simulink model "simulatneously"  (R2015b)
settings: Solver=VariableStepAuto  StartTime=0.0  StopTime=5  RelTol=1e-3
libraries: powerlib x36, powerlib_meascontrol x7, powerlib_extras x7
settings Model: Creator=fujitsu  LastModifiedBy=fujitsu

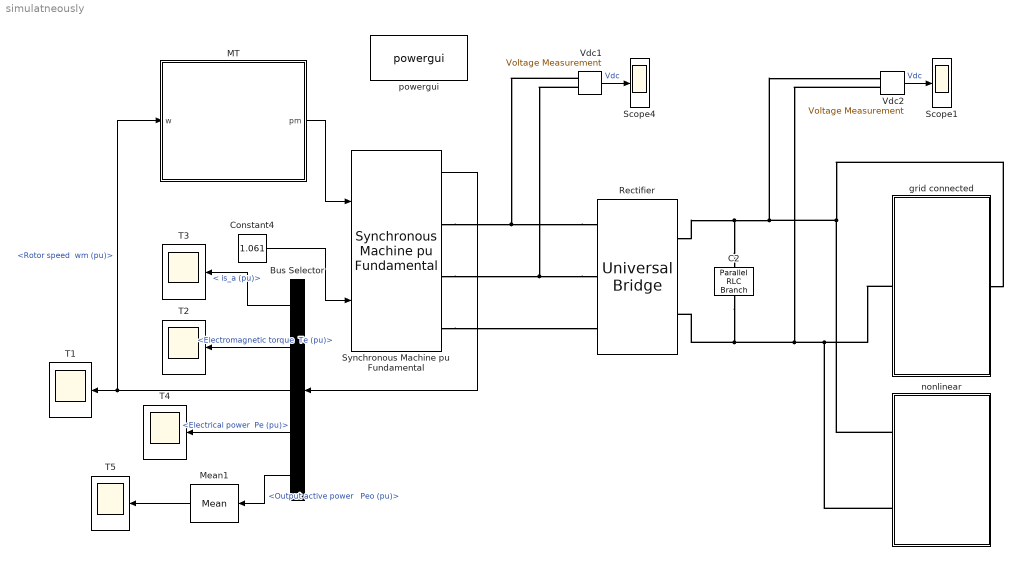
== system simulatneously ==
  Bus Selector : BusSelector  OutputSignals="Stator current. is_a (pu),Mechanical.Electromagnetic torque  Te (pu),Mechanical.Rotor speed  wm (pu),Mechanical.Electrical power  Pe (pu),Output active power   Peo (pu)"
  C2 : powerlib/Elements/Parallel RLC Branch  LConnTagsString=a  RConnTagsString=__new0  BranchType=C  Resistance=inf  Inductance=inf  SetiL0=off  InitialCurrent=0  Capacitance=5000e-05  Setx0=off  InitialVoltage=0  Measurements=None
  Constant4 : Constant  Value=1.061
  MT : Subsystem
  Mean1 : powerlib_meascontrol/Measurements/Mean  Freq=50  Vinit=0  Ts=50e-6
  Rectifier : powerlib/Power Electronics/Universal Bridge  Arms=3  SnubberResistance=50  SnubberCapacitance=0.1e-6  Device=Diodes  Ron=1e-3  Lon=0  ForwardVoltages="[  0.8  0.8  ]"  ForwardVoltage=.7  GTOparameters=[ 10e-6 , 20e-6 ]  IGBTparameters=[ 1e-6 , 2e-6 ]  Measurements=Device currents  Measurements_2=None  converterType=Rectifier
  Scope1 : Scope
  Scope4 : Scope
  Synchronous Machine pu Fundamental : powerlib/Machines/Synchronous Machine pu Fundamental  PresetModel=No  MechanicalLoad=Mechanical power Pm  ShowDetailedParameters=on  RotorType=Salient-pole  Units=per unit fundamental parameters  MeasurementBus=off  NominalParameters="[ 65e3  500 1600]"  Stator="[ 0.2503  0.114  0.6875  0.6875 ]"  Field="[ 1  10e15/(100*pi)]"  Dampers2=[0.0652, 0.5134, 0.0287, 0.2553, 7.765e-3, 0.9167 ]  Dampers1="[ 1.17E-02  0.182  1.97E-02  0.384 ]"  Mechanical=[ 6 0 2]  PolePairs=20  InitialConditions="[ 0  0  0  0  0  0  0  0  1 ]"  SetSaturation=off  Saturation=[0.6404,0.7127,0.8441,0.9214,0.9956,1.082,1.19,1.316,1.457;0.7,0.7698,0.8872,0.9466,0.9969,1.046,1.1,1.151,1.201]  LoadFlowParameters=[1,0,0,0,0]  TsPowergui=0  TsBlock=-1  IterativeModel=Trapezoidal non iterative  BusType=swing  Pref=0  Qref=0  Qmin=-inf  Qmax=inf  PLF=0  QLF=0
  T{1..5} (5 alike) : Scope
  Vdc1 : powerlib/Measurements/Voltage Measurement  Tag=PoWeRsYsTeMmEaSuReMeNt  PhasorSimulation=off  OutputType=Magnitude  PSBequivalent=0
  Vdc2 : powerlib/Measurements/Voltage Measurement  Tag=PoWeRsYsTeMmEaSuReMeNt  PhasorSimulation=off  OutputType=Magnitude  PSBequivalent=0
  grid connected : Subsystem
  nonlinear : Subsystem
  powergui : powerlib/powergui  SimulationMode=Discrete  SolverType=Tustin  SampleTime=5e-6  frequency=60  SPID=off  DisableSnubberDevices=off  DisableRonSwitches=off  DisableVfSwitches=off  SwTol=0  DisplayEquations=off  Interpol=off  ExternalGateDelay=off  methode=off  Ts=0  FunctionMessages=off  echomessages=off  HookPort=off  EnableUseOfTLC=off  x0status=blocks  frequencyindice=0  Pbase=100e6  ErrMax=0.0001  Iterations=50  UnitsV=kV  UnitsW=MW  buscounter=0  RestoreLinks=warning  ResistiveCurrentMeasurement=off  Frange=[0:2:500]  Ylog=off  Xlog=on  ShowGrid=off  save=off  variable=ZData  structure=Vs  ZoomFFT=on  StartTime=1/60  cycles=1  DisplayStyle=1  fundamental=60  FreqAxis=on  MaxFrequency=10000  frequencyindicesteady=1  RmsSteady=1  display=off
  wires:
  MT/1(pm) -> Synchronous Machine pu Fundamental/1
  Synchronous Machine pu Fundamental/1 -> Bus Selector/1
  Bus Selector/1 -> T3/1  "< is_a (pu)>"
  Bus Selector/2 -> T2/1  "<Electromagnetic torque  Te (pu)>"
  Bus Selector/3 -> T1/1, MT/1(w)  "<Rotor speed  wm (pu)>"
  Constant4/1 -> Synchronous Machine pu Fundamental/2
  Vdc1/1 -> Scope4/1  "Vdc"
  Bus Selector/4 -> T4/1  "<Electrical power  Pe (pu)>"
  Bus Selector/5 -> Mean1/1  "<Output active power   Peo (pu)>"
  Mean1/1 -> T5/1
  Vdc2/1 -> Scope1/1  "Vdc"
  connections:
  C2/LConn1 -- Rectifier/RConn1 -- nonlinear/RConn1 -- grid connected/LConn1 -- Vdc2/LConn1
  C2/RConn1 -- Rectifier/RConn2 -- grid connected/RConn1 -- nonlinear/RConn2 -- Vdc2/LConn2
  Rectifier/LConn1 -- Synchronous Machine pu Fundamental/RConn1 -- Vdc1/LConn1
  Rectifier/LConn2 -- Synchronous Machine pu Fundamental/RConn2 -- Vdc1/LConn2
  Synchronous Machine pu Fundamental/RConn3 -- Rectifier/LConn3

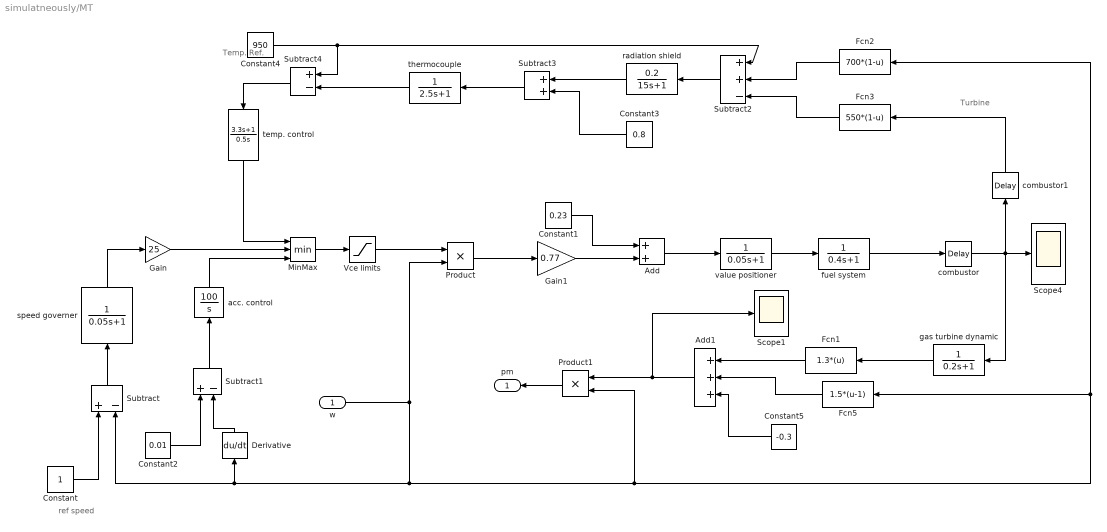
== system simulatneously/MT ==
  note: ref speed
  note: Temp.
      | Ref.
  note: Turbine
  w : Inport
  Add : Sum
  Add1 : Sum  Inputs=+++
  Constant : Constant
  Constant1 : Constant  Value=0.23
  Constant2 : Constant  Value=0.01
  Constant3 : Constant  Value=0.8
  Constant4 : Constant  Value=950
  Constant5 : Constant  Value=-0.3
  Derivative : Derivative  CoefficientInTFapproximation=0.001
  Fcn1 : Fcn  Expr=1.3*(u)
  Fcn2 : Fcn  Expr=700*(1-u)
  Fcn3 : Fcn  Expr=550*(1-u)
  Fcn5 : Fcn  Expr=1.5*(u-1)
  Gain : Gain  Gain=25
  Gain1 : Gain  Gain=0.77
  MinMax : MinMax  Inputs=3
  Product : Product  RndMeth=Zero
  Product1 : Product  RndMeth=Zero
  Scope1 : Scope
  Scope4 : Scope
  Subtract : Sum  Inputs=+-
  Subtract1 : Sum  Inputs=+-
  Subtract2 : Sum  Inputs=++-
  Subtract3 : Sum
  Subtract4 : Sum  Inputs=+-
  Vce limits : Saturate  UpperLimit=1.5  LowerLimit=-0.1
  acc. control : TransferFcn  Numerator=[0 100]  Denominator=[1 0]
  combustor : TransportDelay  DelayTime=0.01
  combustor1 : TransportDelay  DelayTime=0.04
  fuel system : TransferFcn  Denominator=[0.4 1]
  gas turbine dynamic : TransferFcn  Denominator=[0.2 1]
  radiation shield : TransferFcn  Numerator=[0.2]  Denominator=[15 1]
  speed governer : TransferFcn  Numerator=[0 1]  Denominator=[0.05 1]
  temp. control : TransferFcn  Numerator=[3.3 1]  Denominator=[0.5 0]
  thermocouple : TransferFcn  Denominator=[2.5 1]
  value positioner : TransferFcn  Denominator=[0.05 1]
  pm : Outport
  wires:
  Constant/1 -> Subtract/1
  Subtract/1 -> speed governer/1
  Vce limits/1 -> Product/1
  Product/1 -> Gain1/1
  Gain1/1 -> Add/2
  Constant1/1 -> Add/1
  Add/1 -> value positioner/1
  value positioner/1 -> fuel system/1
  fuel system/1 -> combustor/1
  combustor/1 -> gas turbine dynamic/1, combustor1/1, Scope4/1
  Add1/1 -> Scope1/1, Product1/1
  Gain/1 -> MinMax/2
  Derivative/1 -> Subtract1/2
  Constant2/1 -> Subtract1/1
  Subtract1/1 -> acc. control/1
  acc. control/1 -> MinMax/3
  MinMax/1 -> Vce limits/1
  combustor1/1 -> Fcn3/1
  Fcn3/1 -> Subtract2/3
  Fcn2/1 -> Subtract2/2
  radiation shield/1 -> Subtract3/1
  Constant3/1 -> Subtract3/2
  Subtract2/1 -> radiation shield/1
  Subtract3/1 -> thermocouple/1
  thermocouple/1 -> Subtract4/2
  Constant4/1 -> Subtract4/1, Subtract2/1
  Subtract4/1 -> temp. control/1
  temp. control/1 -> MinMax/1
  speed governer/1 -> Gain/1
  w/1 -> Product/2, Product1/2, Fcn2/1, Fcn5/1, Derivative/1, Subtract/2
  gas turbine dynamic/1 -> Fcn1/1
  Fcn1/1 -> Add1/1
  Constant5/1 -> Add1/3
  Fcn5/1 -> Add1/2
  Product1/1 -> pm/1

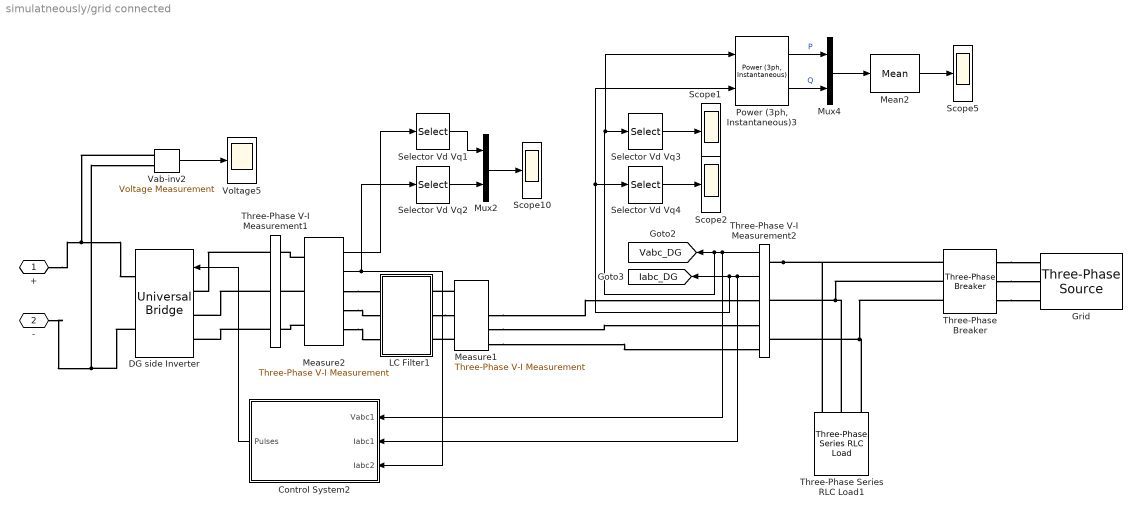
== system simulatneously/grid connected ==
  Control System2 : Subsystem
      mask Display: fprintf('desired performance')
  DG side Inverter : powerlib/Power Electronics/Universal Bridge  Arms=3  SnubberResistance=10000  SnubberCapacitance=inf  Device=IGBT / Diodes  Ron=1e-4  Lon=0  ForwardVoltages="[  1  1  ]"  ForwardVoltage=.8  GTOparameters=[ 10e-6 , 20e-6 ]  IGBTparameters=[ 1e-6 , 2e-6 ]  Measurements=None  Measurements_2=None  converterType=Rectifier
  Grid : powerlib/Electrical Sources/Three-Phase Source  InternalConnection=Yg  VoltagePhases=off  Voltage=380  PhaseAngle=0  Voltage_phases=[25e3 25e3 25e3]/sqrt(3)  PhaseAngles_phases=[0 -120 +120]  Frequency=50  NonIdealSource=on  SpecifyImpedance=off  Resistance=0.02  Inductance=0.3e-3  ShortCircuitLevel=100e6  BaseVoltage=25e3  XRratio=7  BusType=swing  Pref=0  Qref=0  Prefabc=[10e3, 10e3, 10e3]  Qrefabc=[0, 0, 0]  Qmin=-inf  Qmax=inf
  LC Filter1 : Subsystem
  Mean2 : powerlib_meascontrol/Measurements/Mean  Freq=50  Vinit=0  Ts=50e-6
  Measure1 : powerlib/Measurements/Three-Phase V-I Measurement  VoltageMeasurement=phase-to-phase  SetLabelV=off  LabelV=V1  Vpu=off  VpuLL=off  CurrentMeasurement=yes  SetLabelI=off  LabelI=I1  Ipu=off  Pbase=10e3  Vbase=400  OutputType=Magnitude  PhasorSimulation=off  PSBequivalent=0
  Measure2 : powerlib/Measurements/Three-Phase V-I Measurement  VoltageMeasurement=phase-to-phase  SetLabelV=off  LabelV=V1  Vpu=off  VpuLL=on  CurrentMeasurement=yes  SetLabelI=off  LabelI=I1  Ipu=on  Pbase=100e3  Vbase=380  OutputType=Magnitude  PhasorSimulation=off  PSBequivalent=0
  Mux2 : Mux  Inputs=2
  Mux4 : Mux  Inputs=2
  "Power (3ph, Instantaneous)3" : powerlib_meascontrol/Measurements/Power (3ph, Instantaneous)
  Scope{1..2,5,10} (4 alike) : Scope
  Selector Vd Vq{1..4} (4 alike) : Selector  InputPortWidth=3  IndexOptions=Index vector (dialog)  Indices=[1]  OutputSizes=1
  Three-Phase Series RLC Load1 : powerlib/Elements/Three-Phase Series RLC Load  LConnTagsString=A|B|C  Configuration=Y (grounded)  NominalVoltage=380  Vabc=[1e3 1e3 1e3]  Vabcp=[1e3 1e3 1e3]  NominalFrequency=50  UnbalancedPower=off  ActivePower=1e3  InductivePower=0  CapacitivePower=0  Pabc=[10e3 9e3 11e3]  QLabc=[100 90 110]  QCabc=[100 90 110]  Pabcp=[10e3 9e3 11e3]  QLabcp=[100 90 110]  QCabcp=[100 90 110]  Measurements=None  LoadType=constant Z
  Three-Phase V-I Measurement1 : powerlib/Measurements/Three-Phase V-I Measurement  VoltageMeasurement=no  SetLabelV=off  LabelV=Vabc  Vpu=on  VpuLL=off  CurrentMeasurement=no  SetLabelI=off  LabelI=Iabc  Ipu=on  Pbase=300e3  Vbase=208  OutputType=Complex  PhasorSimulation=off  PSBequivalent=0
  Three-Phase V-I Measurement2 : powerlib/Measurements/Three-Phase V-I Measurement  VoltageMeasurement=phase-to-phase  SetLabelV=off  LabelV=Vabc  Vpu=off  VpuLL=on  CurrentMeasurement=yes  SetLabelI=off  LabelI=Iabc  Ipu=on  Pbase=100e3  Vbase=380  OutputType=Complex  PhasorSimulation=off  PSBequivalent=0
  Three-Phase Breaker : powerlib/Elements/Three-Phase Breaker  InitialState=closed  SwitchA=on  SwitchB=on  SwitchC=on  SwitchTimes=[15]  External=off  BreakerResistance=0.01  SnubberResistance=1e6  SnubberCapacitance=inf  Measurements=None
  Vab-inv2 : powerlib/Measurements/Voltage Measurement  Tag=PoWeRsYsTeMmEaSuReMeNt  PhasorSimulation=off  OutputType=Magnitude  PSBequivalent=0
  Voltage5 : Scope
  + : PMIOPort  Port=1  Side=Left
  - : PMIOPort  Port=2  Side=Right
  tag scope: Iabc_DG=global, Vabc_DG=global
  wires:
  Three-Phase V-I Measurement2/1 -> Control System2/1(Vabc1), "Power (3ph, Instantaneous)3"/1, Selector Vd Vq3/1, [Vabc_DG]
  Three-Phase V-I Measurement2/2 -> Control System2/2(Iabc1), "Power (3ph, Instantaneous)3"/2, Selector Vd Vq4/1, [Iabc_DG]
  Vab-inv2/1 -> Voltage5/1
  Mux2/1 -> Scope10/1
  Selector Vd Vq1/1 -> Mux2/1
  Selector Vd Vq2/1 -> Mux2/2
  Measure2/1 -> Selector Vd Vq1/1
  Measure2/2 -> Control System2/3(Iabc2), Selector Vd Vq2/1
  Selector Vd Vq3/1 -> Scope1/1
  Selector Vd Vq4/1 -> Scope2/1
  Mux4/1 -> Mean2/1
  "Power (3ph, Instantaneous)3"/1 -> Mux4/1  "P"
  "Power (3ph, Instantaneous)3"/2 -> Mux4/2  "Q"
  Mean2/1 -> Scope5/1
  Control System2/1(Pulses) -> DG side Inverter/1
  connections:
  DG side Inverter/RConn2 -- -/RConn1 -- Vab-inv2/LConn2
  Vab-inv2/LConn1 -- DG side Inverter/RConn1 -- +/RConn1
  Three-Phase V-I Measurement2/LConn1 -- Three-Phase Breaker/LConn1 -- Three-Phase Series RLC Load1/LConn1
  Three-Phase Series RLC Load1/LConn2 -- Three-Phase Breaker/LConn2 -- Three-Phase V-I Measurement2/LConn2
  Three-Phase Series RLC Load1/LConn3 -- Three-Phase Breaker/LConn3 -- Three-Phase V-I Measurement2/LConn3
  Three-Phase V-I Measurement1/RConn3 -- DG side Inverter/LConn3
  Three-Phase V-I Measurement1/RConn1 -- DG side Inverter/LConn1
  Measure1/RConn1 -- Three-Phase V-I Measurement2/RConn1
  Three-Phase V-I Measurement1/RConn2 -- DG side Inverter/LConn2
  Measure1/RConn3 -- Three-Phase V-I Measurement2/RConn3
  Measure1/LConn1 -- LC Filter1/RConn1
  Three-Phase Breaker/RConn2 -- Grid/RConn2
  Measure1/LConn3 -- LC Filter1/RConn3
  Measure2/LConn2 -- Three-Phase V-I Measurement1/LConn2
  Three-Phase Breaker/RConn1 -- Grid/RConn1
  Measure1/RConn2 -- Three-Phase V-I Measurement2/RConn2
  LC Filter1/RConn2 -- Measure1/LConn2
  Three-Phase Breaker/RConn3 -- Grid/RConn3
  Measure2/RConn3 -- LC Filter1/LConn3
  Measure2/RConn2 -- LC Filter1/LConn2
  Measure2/RConn1 -- LC Filter1/LConn1
  Measure2/LConn3 -- Three-Phase V-I Measurement1/LConn3
  Measure2/LConn1 -- Three-Phase V-I Measurement1/LConn1

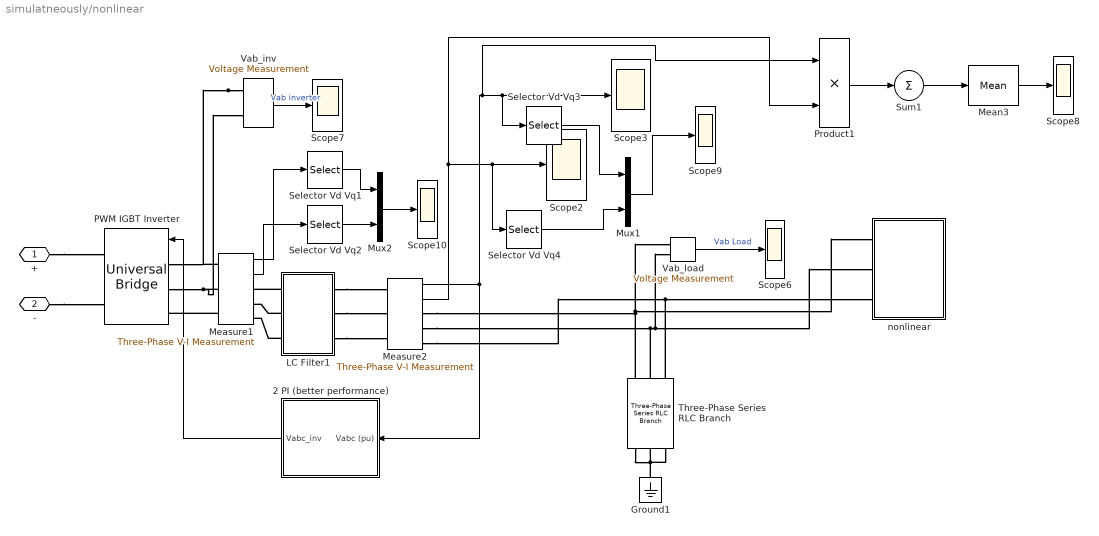
== system simulatneously/nonlinear ==
  2 PI (better performance) : Subsystem  mask{kp=0.01, ki=5}
  Ground1 : powerlib/Elements/Ground  LConnTagsString=a
  LC Filter1 : Subsystem
  Mean3 : powerlib_meascontrol/Measurements/Mean  Freq=50  Vinit=0  Ts=50e-6
  Measure1 : powerlib/Measurements/Three-Phase V-I Measurement  VoltageMeasurement=phase-to-phase  SetLabelV=off  LabelV=V1  Vpu=off  VpuLL=off  CurrentMeasurement=yes  SetLabelI=off  LabelI=I1  Ipu=off  Pbase=10e3  Vbase=400  OutputType=Magnitude  PhasorSimulation=off  PSBequivalent=0
  Measure2 : powerlib/Measurements/Three-Phase V-I Measurement  VoltageMeasurement=phase-to-phase  SetLabelV=off  LabelV=V1  Vpu=off  VpuLL=on  CurrentMeasurement=yes  SetLabelI=off  LabelI=I1  Ipu=on  Pbase=30e3  Vbase=380  OutputType=Magnitude  PhasorSimulation=off  PSBequivalent=0
  Mux1 : Mux  Inputs=2
  Mux2 : Mux  Inputs=2
  PWM IGBT Inverter : powerlib/Power Electronics/Universal Bridge  Arms=3  SnubberResistance=5000  SnubberCapacitance=inf  Device=IGBT / Diodes  Ron=1e-3  Lon=0  ForwardVoltages="[  0.0  0.0  ]"  ForwardVoltage=.8  GTOparameters=[ 1e-6 ,1e-6 ]  IGBTparameters=[ 1e-6 , 2e-6 ]  Measurements=Device currents  Measurements_2=None  converterType=Rectifier
  Product1 : Product  SaturateOnIntegerOverflow=on  InputSameDT=on  OutDataTypeStr=Inherit: Same as first input
  Scope{2..3,6..10} (7 alike) : Scope
  Selector Vd Vq{1..4} (4 alike) : Selector  InputPortWidth=3  IndexOptions=Index vector (dialog)  Indices=[1]  OutputSizes=1
  Sum1 : Sum  Inputs=1  SaturateOnIntegerOverflow=on  InputSameDT=on  OutDataTypeStr=Inherit: Same as first input
  Three-Phase Series RLC Branch : powerlib/Elements/Three-Phase Series RLC Branch  LConnTagsString=A|B|C  RConnTagsString=A|B|C  BranchType=R  Resistance=50  Inductance=1e-3  Capacitance=1e-6  Measurements=None
  Vab_inv : powerlib/Measurements/Voltage Measurement  Tag=PoWeRsYsTeMmEaSuReMeNt  PhasorSimulation=off  OutputType=Magnitude  PSBequivalent=0
  Vab_load : powerlib/Measurements/Voltage Measurement  Tag=PoWeRsYsTeMmEaSuReMeNt  PhasorSimulation=off  OutputType=Magnitude  PSBequivalent=0
  nonlinear : Subsystem
  + : PMIOPort  Port=1  Side=Right
  - : PMIOPort  Port=2  Side=Right
  wires:
  Vab_load/1 -> Scope6/1  "Vab Load"
  Vab_inv/1 -> Scope7/1  "Vab inverter"
  2 PI (better performance)/1(Vabc_inv) -> PWM IGBT Inverter/1
  Measure2/1 -> 2 PI (better performance)/1(Vabc (pu)), Product1/1, Selector Vd Vq3/1, Scope3/1
  Measure2/2 -> Product1/2, Selector Vd Vq4/1, Scope2/1
  Mean3/1 -> Scope8/1
  Mux1/1 -> Scope9/1
  Mux2/1 -> Scope10/1
  Measure1/1 -> Selector Vd Vq1/1
  Selector Vd Vq1/1 -> Mux2/1
  Measure1/2 -> Selector Vd Vq2/1
  Selector Vd Vq2/1 -> Mux2/2
  Sum1/1 -> Mean3/1
  Product1/1 -> Sum1/1
  Selector Vd Vq3/1 -> Mux1/1
  Selector Vd Vq4/1 -> Mux1/2
  connections:
  Measure1/LConn2 -- PWM IGBT Inverter/LConn2 -- Vab_inv/LConn2
  Vab_inv/LConn1 -- PWM IGBT Inverter/LConn1 -- Measure1/LConn1
  Measure2/RConn1 -- Three-Phase Series RLC Branch/LConn1 -- nonlinear/LConn1 -- Vab_load/LConn1
  Measure2/RConn2 -- Three-Phase Series RLC Branch/LConn2 -- nonlinear/LConn2 -- Vab_load/LConn2
  Three-Phase Series RLC Branch/RConn2 -- Three-Phase Series RLC Branch/RConn1 -- Ground1/LConn1 -- Three-Phase Series RLC Branch/RConn3
  LC Filter1/RConn3 -- Measure2/LConn3
  LC Filter1/LConn2 -- Measure1/RConn2
  Measure1/LConn3 -- PWM IGBT Inverter/LConn3
  LC Filter1/RConn1 -- Measure2/LConn1
  LC Filter1/LConn1 -- Measure1/RConn1
  LC Filter1/LConn3 -- Measure1/RConn3
  LC Filter1/RConn2 -- Measure2/LConn2
  +/RConn1 -- PWM IGBT Inverter/RConn1
  -/RConn1 -- PWM IGBT Inverter/RConn2
  Measure2/RConn3 -- Three-Phase Series RLC Branch/LConn3 -- nonlinear/LConn3

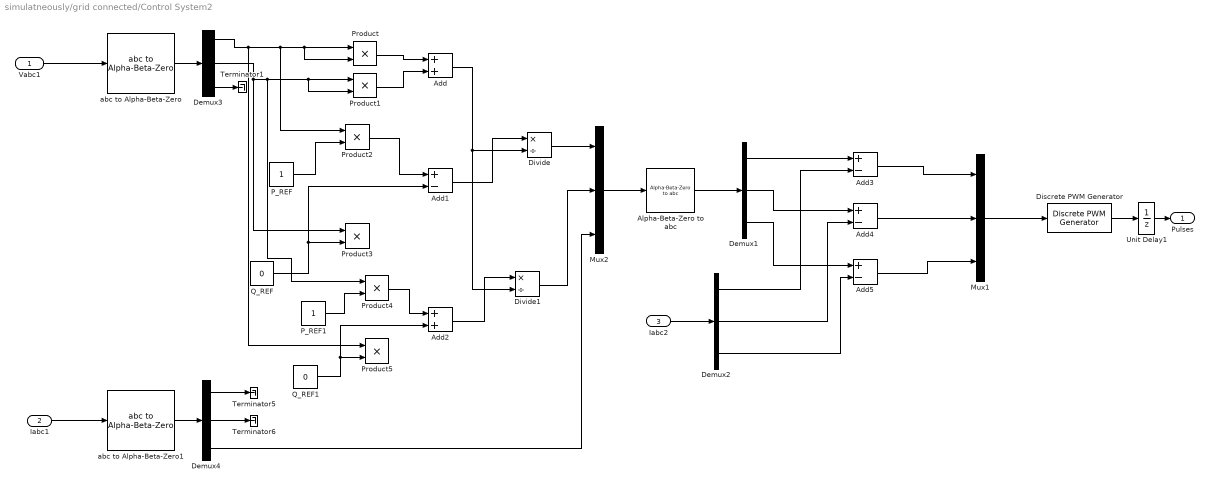
== system simulatneously/grid connected/Control System2 ==
  Vabc1 : Inport  PortDimensions=3
  Iabc1 : Inport  Port=2  PortDimensions=3
  Iabc2 : Inport  Port=3  PortDimensions=3
  Add : Sum
  Add{1,3..5} (4 alike) : Sum  Inputs=+-
  Add2 : Sum
  Alpha-Beta-Zero to abc : powerlib_meascontrol/Transformations/Alpha-Beta-Zero to abc
  Demux{1..4} (4 alike) : Demux  Outputs=3
  Discrete PWM Generator : powerlib_extras/Discrete  Control Blocks/Discrete PWM Generator  GeneratorMode="3-arm  bridge (6 pulses)"  Fc=20000  Ts=5e-6  Internal=off  mIndex=0.4  Freq=60  Phase=0
  Divide : Product  Inputs=*/
  Divide1 : Product  Inputs=*/
  Mux1 : Mux  Inputs=3
  Mux2 : Mux  Inputs=3
  P_REF : Constant
  P_REF1 : Constant
  Product{,1..5} (6 alike) : Product
  Q_REF : Constant  Value=0
  Q_REF1 : Constant  Value=0
  Terminator1 : Terminator
  Terminator5 : Terminator
  Terminator6 : Terminator
  Unit Delay1 : UnitDelay  SampleTime=2e-6
  abc to Alpha-Beta-Zero : powerlib_meascontrol/Transformations/abc to Alpha-Beta-Zero
  abc to Alpha-Beta-Zero1 : powerlib_meascontrol/Transformations/abc to Alpha-Beta-Zero
  Pulses : Outport
  wires:
  Unit Delay1/1 -> Pulses/1
  Discrete PWM Generator/1 -> Unit Delay1/1
  Vabc1/1 -> abc to Alpha-Beta-Zero/1
  abc to Alpha-Beta-Zero/1 -> Demux3/1
  Demux3/1 -> Product/1, Product/2, Product2/1, Product5/1
  Demux3/2 -> Product4/1, Product1/2, Product1/1, Product3/1
  Product/1 -> Add/1
  Product1/1 -> Add/2
  P_REF/1 -> Product2/2
  Q_REF/1 -> Add1/2, Product3/2
  Product2/1 -> Add1/1
  Add1/1 -> Divide/1
  Add/1 -> Divide1/2, Divide/2
  Divide/1 -> Mux2/1
  P_REF1/1 -> Product4/2
  Q_REF1/1 -> Add2/2, Product5/2
  Product4/1 -> Add2/1
  Add2/1 -> Divide1/1
  Divide1/1 -> Mux2/2
  Iabc1/1 -> abc to Alpha-Beta-Zero1/1
  abc to Alpha-Beta-Zero1/1 -> Demux4/1
  Demux4/3 -> Mux2/3
  Demux4/1 -> Terminator5/1
  Demux4/2 -> Terminator6/1
  Mux2/1 -> Alpha-Beta-Zero to abc/1
  Alpha-Beta-Zero to abc/1 -> Demux1/1
  Demux1/1 -> Add3/1
  Iabc2/1 -> Demux2/1
  Demux2/1 -> Add3/2
  Demux1/2 -> Add4/1
  Demux2/2 -> Add4/2
  Demux1/3 -> Add5/1
  Demux2/3 -> Add5/2
  Add3/1 -> Mux1/1
  Add4/1 -> Mux1/2
  Add5/1 -> Mux1/3
  Mux1/1 -> Discrete PWM Generator/1
  Demux3/3 -> Terminator1/1

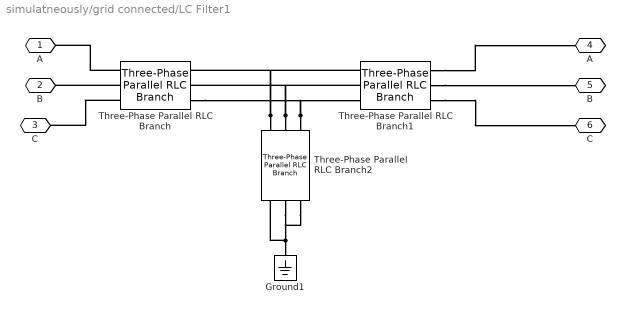
== system simulatneously/grid connected/LC Filter1 ==
  Ground1 : powerlib/Elements/Ground  LConnTagsString=a
  Three-Phase Parallel RLC Branch : powerlib/Elements/Three-Phase Parallel RLC Branch  LConnTagsString=A|B|C  RConnTagsString=A|B|C  BranchType=L  Resistance=1  Inductance=5.7e-3  Capacitance=1e-6  Measurements=None
  Three-Phase Parallel RLC Branch1 : powerlib/Elements/Three-Phase Parallel RLC Branch  LConnTagsString=A|B|C  RConnTagsString=A|B|C  BranchType=R  Resistance=0.00001  Inductance=5.7e-3  Capacitance=1e-6  Measurements=None
  Three-Phase Parallel RLC Branch2 : powerlib/Elements/Three-Phase Parallel RLC Branch  LConnTagsString=A|B|C  RConnTagsString=A|B|C  BranchType=C  Resistance=1  Inductance=5.7e-3  Capacitance=1000e-6  Measurements=None
  A : PMIOPort  Port=1  Side=Left
  B : PMIOPort  Port=2  Side=Left
  C : PMIOPort  Port=3  Side=Left
  "A " : PMIOPort  Port=4  Side=Right
  "B " : PMIOPort  Port=5  Side=Right
  "C " : PMIOPort  Port=6  Side=Right
  connections:
  Ground1/LConn1 -- Three-Phase Parallel RLC Branch2/RConn2 -- Three-Phase Parallel RLC Branch2/RConn1 -- Three-Phase Parallel RLC Branch2/RConn3
  Three-Phase Parallel RLC Branch1/RConn3 -- "C "/RConn1
  Three-Phase Parallel RLC Branch1/RConn2 -- "B "/RConn1
  Three-Phase Parallel RLC Branch1/RConn1 -- "A "/RConn1
  Three-Phase Parallel RLC Branch2/LConn3 -- Three-Phase Parallel RLC Branch1/LConn3 -- Three-Phase Parallel RLC Branch/RConn3
  Three-Phase Parallel RLC Branch2/LConn2 -- Three-Phase Parallel RLC Branch/RConn2 -- Three-Phase Parallel RLC Branch1/LConn2
  Three-Phase Parallel RLC Branch2/LConn1 -- Three-Phase Parallel RLC Branch/RConn1 -- Three-Phase Parallel RLC Branch1/LConn1
  Three-Phase Parallel RLC Branch/LConn3 -- C/RConn1
  Three-Phase Parallel RLC Branch/LConn2 -- B/RConn1
  Three-Phase Parallel RLC Branch/LConn1 -- A/RConn1

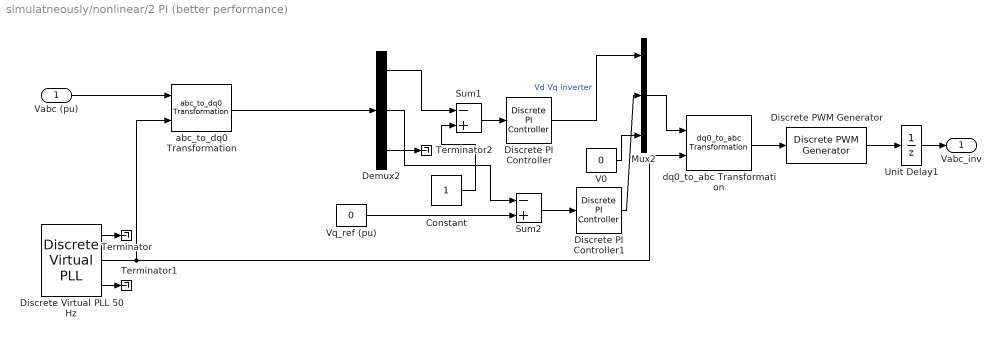
== system simulatneously/nonlinear/2 PI (better performance) ==
  Vabc (pu) : Inport
  Constant : Constant
  Demux2 : Demux  Outputs=3
  Discrete PI Controller : powerlib_extras/Discrete  Control Blocks/Discrete PI Controller  Kp=kp  Ki=ki  Par_Limits=[1 -1]  Init=0  Ts=5e-6
  Discrete PI Controller1 : powerlib_extras/Discrete  Control Blocks/Discrete PI Controller  Kp=kp  Ki=ki  Par_Limits=[1 -1]  Init=0  Ts=5e-6
  Discrete PWM Generator : powerlib_extras/Discrete  Control Blocks/Discrete PWM Generator  GeneratorMode="3-arm  bridge (6 pulses)"  Fc=2000  Ts=5e-6  Internal=off  mIndex=0.4  Freq=60  Phase=0
  Discrete Virtual PLL 50 Hz : powerlib_extras/Discrete  Control Blocks/Discrete Virtual PLL  Freq=50  Phase=0  Ts=5e-6
  Mux2 : Mux  Inputs=3
  Sum1 : Sum  Inputs=-+  SaturateOnIntegerOverflow=on  InputSameDT=on  OutDataTypeStr=Inherit: Same as first input
  Sum2 : Sum  Inputs=-+  SaturateOnIntegerOverflow=on  InputSameDT=on  OutDataTypeStr=Inherit: Same as first input
  Terminator : Terminator
  Terminator1 : Terminator
  Terminator2 : Terminator
  Unit Delay1 : UnitDelay  SampleTime=2e-6
  V0 : Constant  Value=0
  Vq_ref (pu) : Constant  Value=0
  abc_to_dq0 Transformation : powerlib_extras/Measurements/abc_to_dq0 Transformation
  dq0_to_abc Transformation : powerlib_extras/Measurements/dq0_to_abc Transformation
  Vabc_inv : Outport
  wires:
  Vabc (pu)/1 -> abc_to_dq0 Transformation/1
  Demux2/1 -> Sum1/1
  Sum1/1 -> Discrete PI Controller/1
  Mux2/1 -> dq0_to_abc Transformation/1
  Discrete Virtual PLL 50 Hz/2 -> abc_to_dq0 Transformation/2, dq0_to_abc Transformation/2
  Discrete Virtual PLL 50 Hz/1 -> Terminator/1
  Discrete Virtual PLL 50 Hz/3 -> Terminator1/1
  Discrete PWM Generator/1 -> Unit Delay1/1
  dq0_to_abc Transformation/1 -> Discrete PWM Generator/1
  Unit Delay1/1 -> Vabc_inv/1
  abc_to_dq0 Transformation/1 -> Demux2/1
  Demux2/3 -> Terminator2/1
  Constant/1 -> Sum1/2
  Demux2/2 -> Sum2/1
  Vq_ref (pu)/1 -> Sum2/2
  Sum2/1 -> Discrete PI Controller1/1
  Discrete PI Controller/1 -> Mux2/1  "Vd Vq inverter"
  Discrete PI Controller1/1 -> Mux2/2
  V0/1 -> Mux2/3

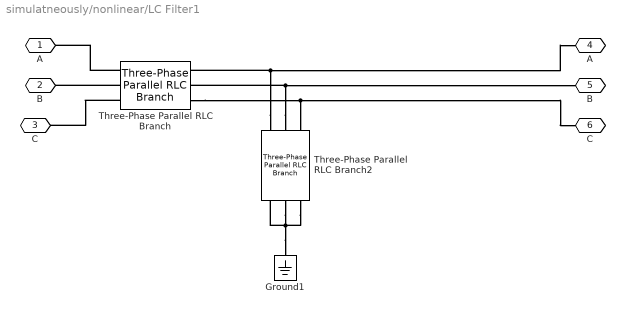
== system simulatneously/nonlinear/LC Filter1 ==
  Ground1 : powerlib/Elements/Ground  LConnTagsString=a
  Three-Phase Parallel RLC Branch : powerlib/Elements/Three-Phase Parallel RLC Branch  LConnTagsString=A|B|C  RConnTagsString=A|B|C  BranchType=L  Resistance=1  Inductance=5.7e-3  Capacitance=1e-6  Measurements=None
  Three-Phase Parallel RLC Branch2 : powerlib/Elements/Three-Phase Parallel RLC Branch  LConnTagsString=A|B|C  RConnTagsString=A|B|C  BranchType=C  Resistance=1  Inductance=5.7e-3  Capacitance=1000e-6  Measurements=None
  A : PMIOPort  Port=1  Side=Left
  B : PMIOPort  Port=2  Side=Left
  C : PMIOPort  Port=3  Side=Left
  "A " : PMIOPort  Port=4  Side=Right
  "B " : PMIOPort  Port=5  Side=Right
  "C " : PMIOPort  Port=6  Side=Right
  connections:
  Ground1/LConn1 -- Three-Phase Parallel RLC Branch2/RConn2 -- Three-Phase Parallel RLC Branch2/RConn1 -- Three-Phase Parallel RLC Branch2/RConn3
  Three-Phase Parallel RLC Branch/RConn3 -- Three-Phase Parallel RLC Branch2/LConn3 -- "C "/RConn1
  Three-Phase Parallel RLC Branch2/LConn2 -- "B "/RConn1 -- Three-Phase Parallel RLC Branch/RConn2
  Three-Phase Parallel RLC Branch2/LConn1 -- "A "/RConn1 -- Three-Phase Parallel RLC Branch/RConn1
  Three-Phase Parallel RLC Branch/LConn3 -- C/RConn1
  Three-Phase Parallel RLC Branch/LConn2 -- B/RConn1
  Three-Phase Parallel RLC Branch/LConn1 -- A/RConn1

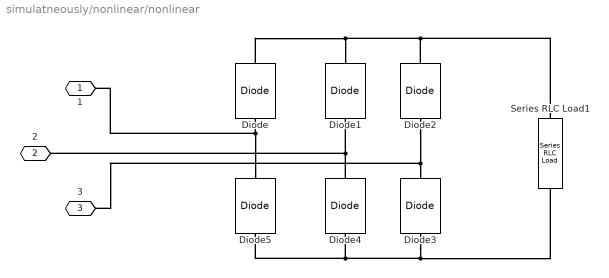
== system simulatneously/nonlinear/nonlinear ==
  Diode{,1..5} (6 alike) : powerlib/Power Electronics/Diode  Ron=0.001  Lon=0  Vf=0.8  IC=0  UseSnubber=off  Rs=500  Cs=250e-9  Measurements=off
  Series RLC Load1 : powerlib/Elements/Series RLC Load  LConnTagsString=a  RConnTagsString=__new0  NominalVoltage=350  NominalFrequency=60  ActivePower=500  InductivePower=100  CapacitivePower=0  Setx0=off  InitialVoltage=0  SetiL0=off  InitialCurrent=0  Measurements=None  LoadType=constant Z
  1 : PMIOPort  Port=1  Side=Left
  2 : PMIOPort  Port=2  Side=Left
  3 : PMIOPort  Port=3  Side=Left
  connections:
  Diode/LConn1 -- 1/RConn1 -- Diode5/RConn1
  Series RLC Load1/LConn1 -- Diode/RConn1 -- Diode1/RConn1 -- Diode2/RConn1
  Diode1/LConn1 -- 2/RConn1 -- Diode4/RConn1
  Diode3/RConn1 -- Diode2/LConn1 -- 3/RConn1
  Diode5/LConn1 -- Diode4/LConn1 -- Diode3/LConn1 -- Series RLC Load1/RConn1
